simulink model "q1_4"  (R2019a)
settings: Solver=FixedStepAuto  StartTime=0.0  StopTime=0.01  FixedStep=1e-7  RelTol=1e-3
libraries: dsparch4 x1
settings Model: Creator=marco  LastModifiedBy=marco

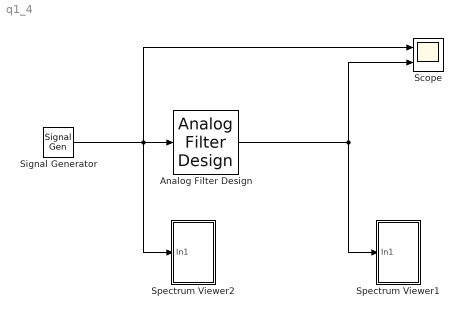
== system q1_4 ==
  Analog Filter Design : dsparch4/Analog Filter Design  method=Butterworth  filttype=Lowpass  N=3  Wlo=2*pi*2e6  Whi=80  Rp=2  Rs=40
  Scope : Scope  NumInputPorts=2
  Signal Generator : SignalGenerator  WaveForm=square  Amplitude=0.2  Frequency=1e5
  Spectrum Viewer1 : Subsystem
  Spectrum Viewer2 : Subsystem
  wires:
  Signal Generator/1 -> Spectrum Viewer2/1(In1), Scope/1, Analog Filter Design/1
  Analog Filter Design/1 -> Spectrum Viewer1/1(In1), Scope/2

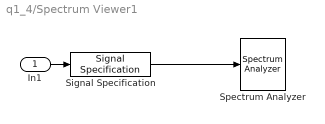
== system q1_4/Spectrum Viewer1 ==
  In1 : Inport
  Signal Specification : SignalSpecification  SampleTime=1e-7
  Spectrum Analyzer : SpectrumAnalyzer
  wires:
  In1/1 -> Signal Specification/1
  Signal Specification/1 -> Spectrum Analyzer/1

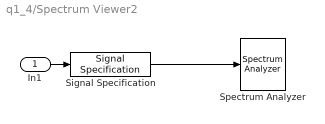
== system q1_4/Spectrum Viewer2 ==
  In1 : Inport
  Signal Specification : SignalSpecification  SampleTime=1e-7
  Spectrum Analyzer : SpectrumAnalyzer
  wires:
  In1/1 -> Signal Specification/1
  Signal Specification/1 -> Spectrum Analyzer/1
